simulink model "es6"  (R2022b)
settings: Solver=VariableStepAuto  StartTime=0.0  StopTime=2  RelTol=1e-3
settings Model: Creator=adlercohen  LastModifiedBy=adlercohen

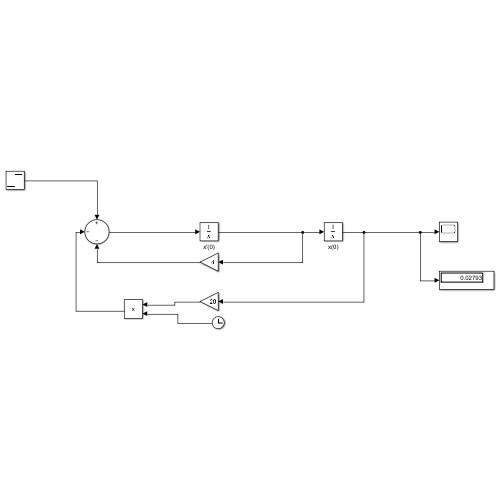
[thumbnail: Simulink's stored preview of the top-level diagram]
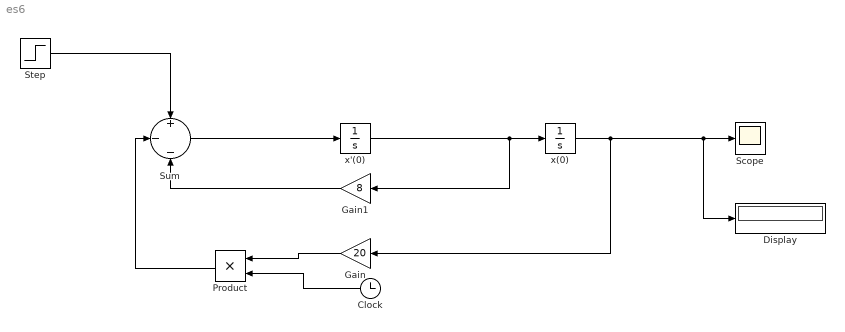
== system es6 ==
  Clock : Clock
  Display : Display
  Gain : Gain  Gain=20
  Gain1 : Gain  Gain=8
  Product : Product
  Scope : Scope
  Step : Step  Time=0  SampleTime=0
  Sum : Sum  Inputs=+|-|-
  x'(0) : Integrator
  x(0) : Integrator
  wires:
  x(0)/1 -> Scope/1, Display/1, Gain/1
  x'(0)/1 -> Gain1/1, x(0)/1
  Product/1 -> Sum/2
  Step/1 -> Sum/1
  Gain1/1 -> Sum/3
  Sum/1 -> x'(0)/1
  Clock/1 -> Product/2
  Gain/1 -> Product/1
